simulink library "FMLibrary_v2"  (R2016b)
settings: Solver=ode45  StartTime=0.0  StopTime=10.0  RelTol=1e-3
undefined symbols (not defined in the file or in its folder): ActuatorStruct, drivePeakCurrent, IdxJoint, JointPositionGuardMax_rad, JointPositionGuardMin_rad, Lb, Lf, Lu, motorTorqueConstant, RobotStruct, sampleTime, transmissionRatio
undefined symbols (not defined in the file): JointAbsoluteEncoderCounts_rev
libraries: simulink x23, VariousBlocksLibrary x10, FM_Library x8, FMLibrary_v2 x5, simulink_extras x1
(part 1 of 2)
settings Model: Creator=niekbeckers  LastModifiedBy=niekbeckers
settings DataIOCC: LimitDataPoints=on  SaveFormat=Array
settings OptimizationCC: BlockReduction=off  BooleanDataType=off  LifeSpan=inf
settings DebuggingCC: SaveWithParameterizedLinksMsg=none  UnderspecifiedInitializationDetection=Classic  MergeDetectMultiDrivingBlocksExec=none  SignalResolutionControl=TryResolveAllWithWarning  StrictBusMsg=Warning  SFUnexpectedBacktrackingDiag=warning  SFNoUnconditionalDefaultTransitionDiag=warning  SFExecutionAtInitializationDiag=none
settings HardwareCC: ProdBitPerPointer=32  ProdBitPerSizeT=32  ProdBitPerPtrDiffT=32  ProdLargestAtomicFloat=None  ProdIntDivRoundTo=Undefined  ProdEndianess=Unspecified  ProdWordSize=32  ProdHWDeviceType=32-bit Generic  TargetUnknown=on
settings ModelReferenceCC: PropagateSignalLabelsOutOfModel=off
settings GRTTargetCC: TargetLangStandard=C89/C90 (ANSI)  GeneratePreprocessorConditionals=Disable all
settings ConfigComp: CovMetricSettings=dw  CovHtmlReporting=on  CovSaveCumulativeToWorkspaceVar=on  CovSaveSingleToWorkspaceVar=on  CovExternalEMLEnable=off  CovSFcnEnable=off

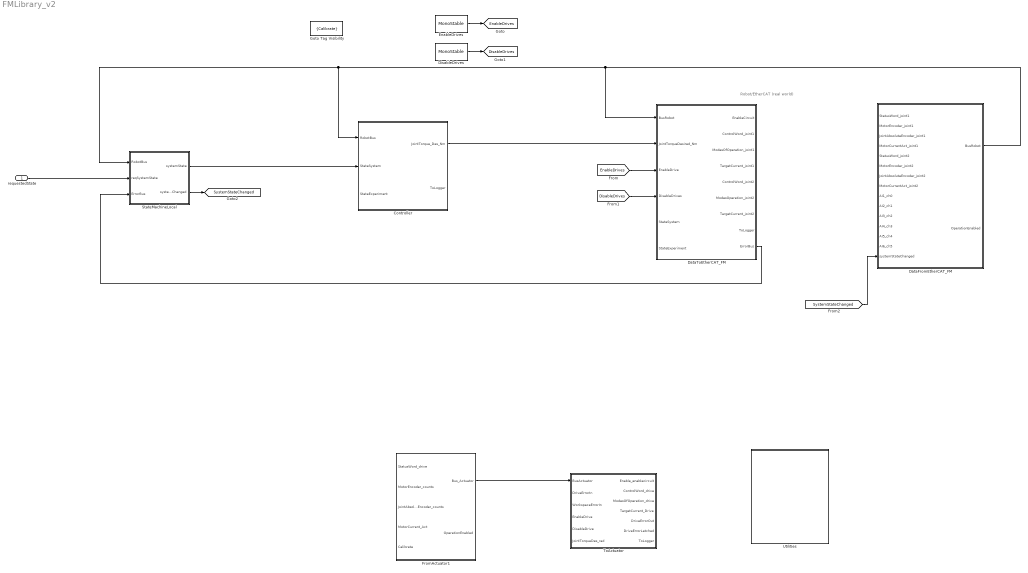
== system FMLibrary_v2 ==
  note: Robot/EtherCAT (real world)
  requestedState : Inport
  Controller : Subsystem
  DataFromEtherCAT_FM : Subsystem
  DataToEtherCAT_FM : Subsystem
  DisableDrives : FM_Library/MonoStable  Value=0  OutMin=[]  OutMax=[]  OutDataTypeStr=Inherit: Inherit from 'Constant value'
  EnableDrives : FM_Library/MonoStable  Value=0  OutMin=[]  OutMax=[]  OutDataTypeStr=Inherit: Inherit from 'Constant value'
  FromActuator1 : Subsystem  mask{ActuatorStruct=RobotStruct.ActuatorStruct}
      mask prompts: ActuatorStruct "Actuator Struct"
  Goto Tag Visibility : GotoTagVisibility  GotoTag=Calibrate
  StateMachineLocal : Subsystem
  ToActuator : Subsystem  mask{ActuatorStruct=RobotStruct.Actuator1}
      mask prompts: ActuatorStruct "Actuator Struct"
  Utilities : Subsystem
  tag scope: DisableDrives=global, EnableDrives=global, SystemStateChanged=global
  wires:
  FromActuator1/1(Bus_Actuator) -> ToActuator/1(BusActuator)
  [EnableDrives] -> DataToEtherCAT_FM/3(EnableDrive)
  [DisableDrives] -> DataToEtherCAT_FM/4(DisableDrives)
  DisableDrives/1 -> [DisableDrives]
  EnableDrives/1 -> [EnableDrives]
  Controller/1(JointTorque_Des_Nm) -> DataToEtherCAT_FM/2(JointTorqueDesired_Nm)
  requestedState/1 -> StateMachineLocal/2(reqSystemState)
  StateMachineLocal/1(systemState) -> Controller/2(StateSystem)
  DataFromEtherCAT_FM/1(BusRobot) -> DataToEtherCAT_FM/1(BusRobot), Controller/1(RobotBus), StateMachineLocal/1(RobotBus)
  DataToEtherCAT_FM/9(ErrorBus) -> StateMachineLocal/3(ErrorBus)
  StateMachineLocal/2(systemStateChanged) -> [SystemStateChanged]
  [SystemStateChanged] -> DataFromEtherCAT_FM/15(systemStateChanged)

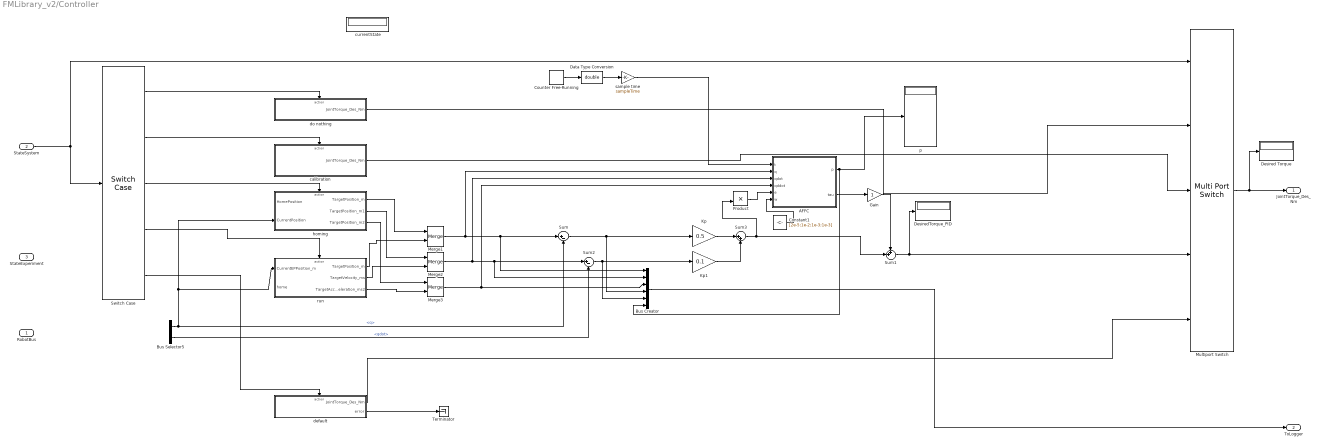
== system FMLibrary_v2/Controller ==
  RobotBus : Inport
  StateSystem : Inport  Port=2
  StateExperiment : Inport  Port=3
  AFFC : MATLAB Function  TreatAsAtomicUnit=on
  Bus Creator : BusCreator  Inputs=6
  Bus Selector5 : BusSelector  OutputSignals=q,qdot
  Constant1 : Constant  Value=[2e-5;1e-2;1e-3;1e-3]
  Counter Free-Running : simulink/Sources/Counter Free-Running  NumBits=32  tsamp=-1
  Data Type Conversion : DataTypeConversion  OutDataTypeStr=double
  Desired Torque : Display
  DesiredTorque_PID : Display
  Gain : Gain
  Kp : Gain  Gain=0.5
  Kp1 : Gain  Gain=0.1
  Merge1 : Merge  InitialOutput=[0;0]
  Merge2 : Merge  InitialOutput=[0;0]
  Merge3 : Merge  InitialOutput=[0;0]
  Multiport Switch : MultiPortSwitch  DataPortOrder=Specify indices  Inputs=4  DataPortIndices={[0,1,201,202,-1],[2],[3,301,4],5}
  Product : Product
  Sum : Sum  Inputs=|+-
  Sum1 : Sum  Inputs=++|
  Sum2 : Sum  Inputs=|+-
  Sum3 : Sum  Inputs=|++
  Switch Case : SwitchCase  CaseConditions={[0,1,201,202,-1],[2],[3,301],4}
  Terminator : Terminator
  calibration : Subsystem  TreatAsAtomicUnit=on
  currentState : Display
  default : Subsystem  TreatAsAtomicUnit=on
  do nothing : Subsystem  TreatAsAtomicUnit=on
  homing : Subsystem
  p : Display
  run : Subsystem
  sample time : Gain  Gain=sampleTime
  JointTorque_Des_Nm : Outport
  ToLogger : Outport  Port=2
  wires:
  Switch Case/2 -> calibration/Action
  Switch Case/1 -> do nothing/Action
  do nothing/1(JointTorque_Des_Nm) -> Multiport Switch/2
  calibration/1(JointTorque_Des_Nm) -> Multiport Switch/3
  default/1(JointTorque_Des_Nm) -> Multiport Switch/5
  Switch Case/5 -> default/Action
  Multiport Switch/1 -> Desired Torque/1, JointTorque_Des_Nm/1
  Switch Case/4 -> run/Action
  Sum/1 -> Bus Creator/4, Kp/1
  homing/1(TargetPosition_m) -> Merge1/1
  Merge1/1 -> AFFC/2(q), Bus Creator/1, Sum/1
  run/1(TargetPosition_m) -> Merge1/2
  Switch Case/3 -> homing/Action
  StateSystem/1 -> Multiport Switch/1, Switch Case/1
  Bus Selector5/1 -> run/1(CurrentEPPosition_m), homing/2(CurrentPosition), Sum/2  "<q>"
  Sum3/1 -> Product/2, Sum1/2
  Sum1/1 -> DesiredTorque_PID/1, Multiport Switch/4
  Gain/1 -> Sum1/1
  run/2(TargetVelocity_ms) -> Merge2/2
  Sum2/1 -> Kp1/1, Bus Creator/5
  Bus Selector5/2 -> Sum2/2  "<qdot>"
  run/3(TargetAcceleration_ms2) -> Merge3/2
  homing/2(TargetPosition_m1) -> Merge2/1
  Merge2/1 -> AFFC/3(qdot), Bus Creator/2, Sum2/1
  homing/3(TargetPosition_m2) -> Merge3/1
  Merge3/1 -> AFFC/4(qddot), Bus Creator/3
  Bus Creator/1 -> ToLogger/1
  default/2(error) -> Terminator/1
  Kp/1 -> Sum3/1
  Kp1/1 -> Sum3/2
  AFFC/1(p) -> Bus Creator/6, p/1
  Data Type Conversion/1 -> sample time/1
  Counter Free-Running/1 -> Data Type Conversion/1
  sample time/1 -> AFFC/1(t)
  Product/1 -> AFFC/5(e)
  Constant1/1 -> AFFC/6(w)
  AFFC/2(tau) -> Gain/1

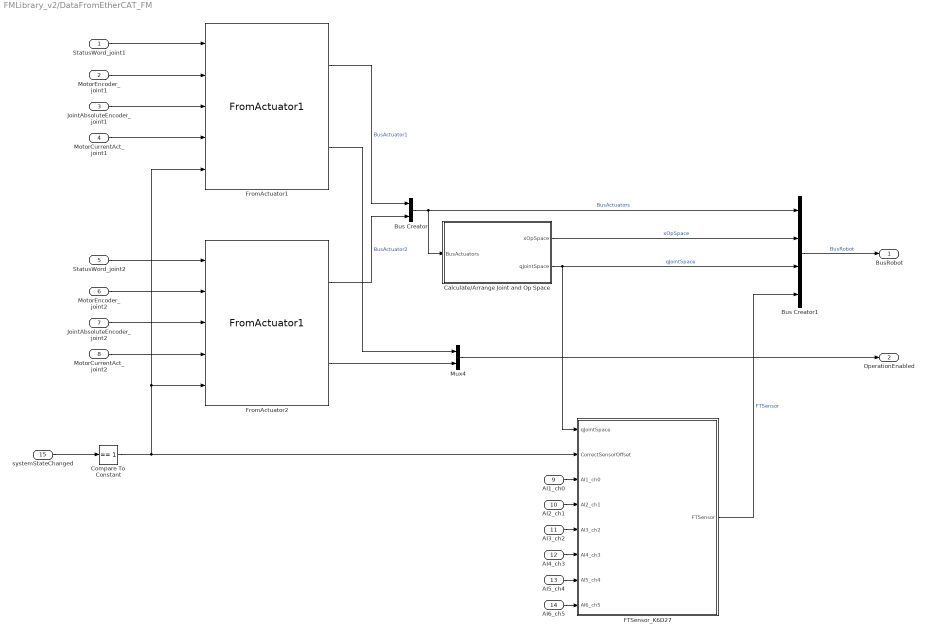
== system FMLibrary_v2/DataFromEtherCAT_FM ==
  StatusWord_joint1 : Inport
  MotorEncoder_joint1 : Inport  Port=2
  JointAbsoluteEncoder_joint1 : Inport  Port=3
  MotorCurrentAct_joint1 : Inport  Port=4
  StatusWord_joint2 : Inport  Port=5
  MotorEncoder_joint2 : Inport  Port=6
  "JointAbsoluteEncoder_joint2 " : Inport  Port=7
  MotorCurrentAct_joint2 : Inport  Port=8
  AI1_ch0 : Inport  Port=9  OutDataTypeStr=int16
  AI2_ch1 : Inport  Port=10  OutDataTypeStr=int16
  AI3_ch2 : Inport  Port=11  OutDataTypeStr=int16
  AI4_ch3 : Inport  Port=12  OutDataTypeStr=int16
  AI5_ch4 : Inport  Port=13  OutDataTypeStr=int16
  AI6_ch5 : Inport  Port=14  OutDataTypeStr=int16
  systemStateChanged : Inport  Port=15
  Bus Creator : BusCreator  Inputs=2
  Bus Creator1 : BusCreator  Inputs=4
  Calculate/Arrange Joint and Op Space : Subsystem
  Compare To Constant : simulink/Logic and Bit Operations/Compare To Constant  relop===  const=1  OutDataTypeStr=boolean
  FTSensor_K6D27 : Subsystem  mask{FTSensorStruct=RobotStruct.FTSensor}
      mask prompts: FTSensorStruct "Struct for force torque sensor"
  FromActuator1 : FMLibrary_v2/Utilities/FromActuator1  ActuatorStruct=RobotStruct.ActuatorStruct
  FromActuator2 : FMLibrary_v2/Utilities/FromActuator1  ActuatorStruct=RobotStruct.ActuatorStruct
  Mux4 : Mux  Inputs=2
  BusRobot : Outport
  OperationEnabled : Outport  Port=2
  wires:
  FromActuator1/1 -> Bus Creator/1  "BusActuator1"
  FromActuator2/1 -> Bus Creator/2  "BusActuator2"
  FromActuator1/2 -> Mux4/1
  Mux4/1 -> OperationEnabled/1
  FromActuator2/2 -> Mux4/2
  MotorEncoder_joint1/1 -> FromActuator1/2
  StatusWord_joint1/1 -> FromActuator1/1
  JointAbsoluteEncoder_joint1/1 -> FromActuator1/3
  MotorCurrentAct_joint1/1 -> FromActuator1/4
  MotorEncoder_joint2/1 -> FromActuator2/2
  StatusWord_joint2/1 -> FromActuator2/1
  "JointAbsoluteEncoder_joint2 "/1 -> FromActuator2/3
  MotorCurrentAct_joint2/1 -> FromActuator2/4
  Bus Creator/1 -> Calculate/Arrange Joint and Op Space/1(BusActuators), Bus Creator1/1  "BusActuators"
  Bus Creator1/1 -> BusRobot/1  "BusRobot"
  Calculate/Arrange Joint and Op Space/1(xOpSpace) -> Bus Creator1/2  "xOpSpace"
  Calculate/Arrange Joint and Op Space/2(qJointSpace) -> FTSensor_K6D27/1(qJointSpace), Bus Creator1/3  "qJointSpace"
  systemStateChanged/1 -> Compare To Constant/1
  AI1_ch0/1 -> FTSensor_K6D27/3(AI1_ch0)
  AI2_ch1/1 -> FTSensor_K6D27/4(AI2_ch1)
  AI3_ch2/1 -> FTSensor_K6D27/5(AI3_ch2)
  AI4_ch3/1 -> FTSensor_K6D27/6(AI4_ch3)
  AI5_ch4/1 -> FTSensor_K6D27/7(AI5_ch4)
  AI6_ch5/1 -> FTSensor_K6D27/8(AI6_ch5)
  FTSensor_K6D27/1(FTSensor) -> Bus Creator1/4  "FTSensor"
  Compare To Constant/1 -> FromActuator2/5, FromActuator1/5, FTSensor_K6D27/2(CorrectSensorOffset)

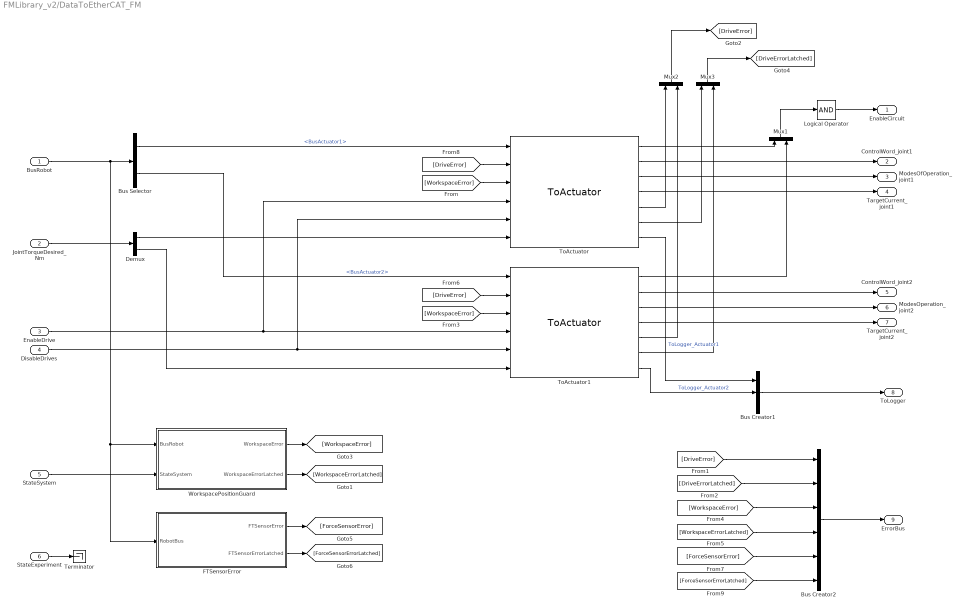
== system FMLibrary_v2/DataToEtherCAT_FM ==
  BusRobot : Inport
  JointTorqueDesired_Nm : Inport  Port=2
  EnableDrive : Inport  Port=3
  DisableDrives : Inport  Port=4
  StateSystem : Inport  Port=5
  StateExperiment : Inport  Port=6
  Bus Creator1 : BusCreator  Inputs=3
  Bus Creator2 : BusCreator  Inputs=6
  Bus Selector : BusSelector  OutputSignals=BusActuators.BusActuator1,BusActuators.BusActuator2
  Demux : Demux  Outputs=2
  FTSensorError : Subsystem
  Logical Operator : Logic  Inputs=1  AllPortsSameDT=off  OutDataTypeStr=boolean
  Mux1 : Mux  Inputs=2
  Mux2 : Mux  Inputs=2
  Mux3 : Mux  Inputs=2
  Terminator : Terminator
  ToActuator : FMLibrary_v2/ToActuator  ActuatorStruct=RobotStruct.Actuator1
  ToActuator1 : FMLibrary_v2/ToActuator  ActuatorStruct=RobotStruct.Actuator1
  WorkspacePositionGuard : Subsystem
  EnableCircuit : Outport
  ControlWord_joint1 : Outport  Port=2
  ModesOfOperation_joint1 : Outport  Port=3
  TargetCurrent_joint1 : Outport  Port=4
  ControlWord_joint2 : Outport  Port=5
  ModesOperation_joint2 : Outport  Port=6
  TargetCurrent_joint2 : Outport  Port=7
  ToLogger : Outport  Port=8
  ErrorBus : Outport  Port=9
  wires:
  ToActuator/5 -> Mux2/1
  ToActuator1/5 -> Mux2/2
  Mux2/1 -> [DriveError]
  ToActuator/6 -> Mux3/1
  ToActuator1/6 -> Mux3/2
  [DriveError] -> ToActuator/2
  Mux1/1 -> Logical Operator/1
  ToActuator/1 -> Mux1/1
  ToActuator1/1 -> Mux1/2
  ToActuator/2 -> ControlWord_joint1/1
  ToActuator/3 -> ModesOfOperation_joint1/1
  ToActuator1/2 -> ControlWord_joint2/1
  ToActuator/4 -> TargetCurrent_joint1/1
  ToActuator1/4 -> TargetCurrent_joint2/1
  ToActuator1/3 -> ModesOperation_joint2/1
  Logical Operator/1 -> EnableCircuit/1
  ToActuator/7 -> Bus Creator1/1  "ToLogger_Actuator1"
  Demux/2 -> ToActuator1/6
  JointTorqueDesired_Nm/1 -> Demux/1
  Demux/1 -> ToActuator/6
  BusRobot/1 -> FTSensorError/1(RobotBus), WorkspacePositionGuard/1(BusRobot), Bus Selector/1
  Bus Selector/2 -> ToActuator1/1  "<BusActuator2>"
  Bus Selector/1 -> ToActuator/1  "<BusActuator1>"
  Bus Creator1/1 -> ToLogger/1
  ToActuator1/7 -> Bus Creator1/2  "ToLogger_Actuator2"
  WorkspacePositionGuard/2(WorkspaceErrorLatched) -> [WorkspaceErrorLatched]
  WorkspacePositionGuard/1(WorkspaceError) -> [WorkspaceError]
  [WorkspaceError] -> ToActuator/3
  DisableDrives/1 -> ToActuator/5, ToActuator1/5
  EnableDrive/1 -> ToActuator/4, ToActuator1/4
  [DriveError] -> ToActuator1/2
  [WorkspaceError] -> ToActuator1/3
  Mux3/1 -> [DriveErrorLatched]
  Bus Creator2/1 -> ErrorBus/1
  [DriveError] -> Bus Creator2/1
  [DriveErrorLatched] -> Bus Creator2/2
  [WorkspaceError] -> Bus Creator2/3
  [WorkspaceErrorLatched] -> Bus Creator2/4
  StateSystem/1 -> WorkspacePositionGuard/2(StateSystem)
  FTSensorError/1(FTSensorError) -> [ForceSensorError]
  FTSensorError/2(FTSensorErrorLatched) -> [ForceSensorErrorLatched]
  [ForceSensorError] -> Bus Creator2/5
  [ForceSensorErrorLatched] -> Bus Creator2/6
  StateExperiment/1 -> Terminator/1

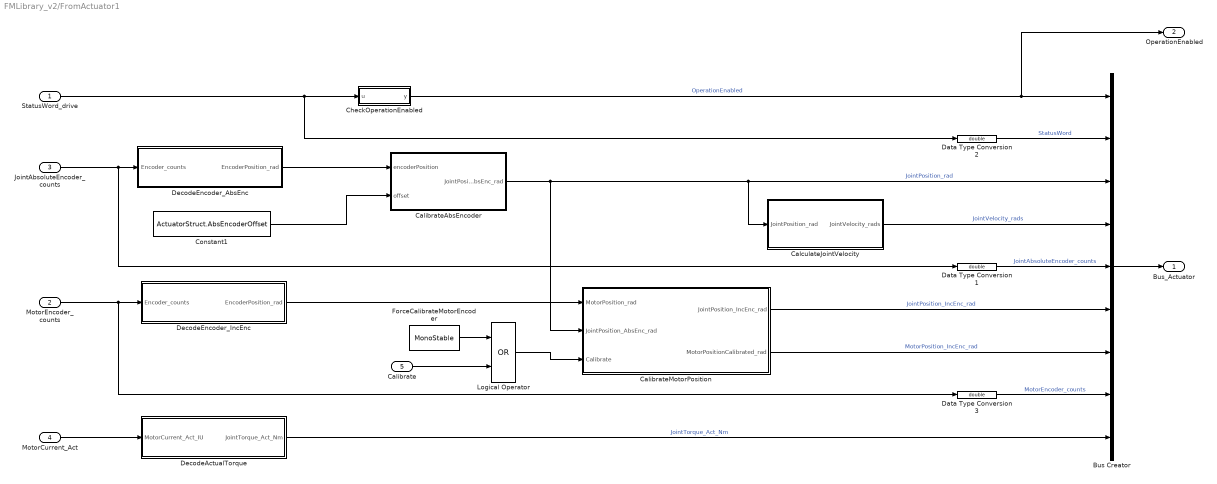
== system FMLibrary_v2/FromActuator1 ==
  StatusWord_drive : Inport
  MotorEncoder_counts : Inport  Port=2
  JointAbsoluteEncoder_counts : Inport  Port=3
  MotorCurrent_Act : Inport  Port=4
  Calibrate : Inport  Port=5
  Bus Creator : BusCreator  Inputs=9
  CalculateJointVelocity : Subsystem
  CalibrateAbsEncoder : MATLAB Function  TreatAsAtomicUnit=on
  "CalibrateMotorPosition    " : MATLAB Function  TreatAsAtomicUnit=on  mask{gearboxRatio=ActuatorStruct.transmissionRatio}
      mask prompts: gearboxRatio "Transmission ratio (e.g. -8) [-]"
  CheckOperationEnabled : MATLAB Function  TreatAsAtomicUnit=on
  Constant1 : Constant  Value=ActuatorStruct.AbsEncoderOffset
  Data Type Conversion1 : DataTypeConversion  OutDataTypeStr=double
  Data Type Conversion2 : DataTypeConversion  OutDataTypeStr=double
  Data Type Conversion3 : DataTypeConversion  OutDataTypeStr=double
  DecodeActualTorque : MATLAB Function  TreatAsAtomicUnit=on  mask(DecodeActualTorque){transmissionRatio=ActuatorStruct.transmissionRatio, motorTorqueConstant=ActuatorStruct.motorTorqueConstant, drivePeakCurrent=ActuatorStruct.drivePeakCurrent}
      mask prompts: transmissionRatio "Transmission ratio (e.g. -8) [-]"; motorTorqueConstant "Motor torque constant [Nm/A]"; drivePeakCurrent "Motor drive peak current Ipeak [A]"
      mask help:
      | Decode Actual Torque value returned from the actuator (motor drive and motor) to torque on the joint (after transmission).
      |
      | Note: due to the way the transmission is set up and the positive motor axis (clockwise is positive as seen from the motor front), there is no need to account for sign change in motor torque or encoder position.
  DecodeEncoder_AbsEnc : MATLAB Function  TreatAsAtomicUnit=on  mask(DecodeEncoder){EncoderCounts_rev=ActuatorStruct.JointAbsoluteEncoderCounts_rev}
      mask prompts: EncoderCounts_rev "Motor encoder increments per revolution (e.g., 8192)"
      mask help: Decode the encoder counts to encoder position in radians
  DecodeEncoder_IncEnc : MATLAB Function  TreatAsAtomicUnit=on  mask(DecodeEncoder){EncoderCounts_rev=ActuatorStruct.MotorEncoderCounts_rev}
      mask prompts: EncoderCounts_rev "Motor encoder increments per revolution (e.g., 8192)"
      mask help: Decode the encoder counts to encoder position in radians
  ForceCalibrateMotorEncoder : FM_Library/MonoStable  Value=0  OutMin=[]  OutMax=[]  OutDataTypeStr=Inherit: Inherit from 'Constant value'
  Logical Operator : Logic  Operator=OR  AllPortsSameDT=off  OutDataTypeStr=boolean
  Bus_Actuator : Outport
  OperationEnabled : Outport  Port=2
  wires:
  Calibrate/1 -> Logical Operator/2
  CalculateJointVelocity/1(JointVelocity_rads) -> Bus Creator/4  "JointVelocity_rads"
  DecodeEncoder_AbsEnc/1(EncoderPosition_rad) -> CalibrateAbsEncoder/1(encoderPosition)
  "CalibrateMotorPosition    "/2(MotorPositionCalibrated_rad) -> Bus Creator/7  "MotorPosition_IncEnc_rad"
  DecodeActualTorque/1(JointTorque_Act_Nm) -> Bus Creator/9  "JointTorque_Act_Nm"
  StatusWord_drive/1 -> Data Type Conversion2/1, CheckOperationEnabled/1(u)
  DecodeEncoder_IncEnc/1(EncoderPosition_rad) -> "CalibrateMotorPosition    "/1(MotorPosition_rad)
  MotorCurrent_Act/1 -> DecodeActualTorque/1(MotorCurrent_Act_IU)
  CheckOperationEnabled/1(y) -> OperationEnabled/1, Bus Creator/1  "OperationEnabled"
  JointAbsoluteEncoder_counts/1 -> Data Type Conversion1/1, DecodeEncoder_AbsEnc/1(Encoder_counts)
  "CalibrateMotorPosition    "/1(JointPosition_IncEnc_rad) -> Bus Creator/6  "JointPosition_IncEnc_rad"
  Data Type Conversion1/1 -> Bus Creator/5  "JointAbsoluteEncoder_counts"
  Data Type Conversion2/1 -> Bus Creator/2  "StatusWord"
  CalibrateAbsEncoder/1(JointPosition_AbsEnc_rad) -> "CalibrateMotorPosition    "/2(JointPosition_AbsEnc_rad), CalculateJointVelocity/1(JointPosition_rad), Bus Creator/3  "JointPosition_rad"
  MotorEncoder_counts/1 -> DecodeEncoder_IncEnc/1(Encoder_counts), Data Type Conversion3/1
  Data Type Conversion3/1 -> Bus Creator/8  "MotorEncoder_counts"
  Bus Creator/1 -> Bus_Actuator/1
  Logical Operator/1 -> "CalibrateMotorPosition    "/3(Calibrate)
  Constant1/1 -> CalibrateAbsEncoder/2(offset)
  ForceCalibrateMotorEncoder/1 -> Logical Operator/1

== system FMLibrary_v2/StateMachineLocal ==
  RobotBus : Inport
  reqSystemState : Inport  Port=2
  ErrorBus : Inport  Port=3
  Bus Selector : BusSelector  OutputSignals=xOpSpace.x,xOpSpace.xdot
  Constant : Constant  Value=RobotStruct.HomeLocationSize
  Constant1 : Constant  Value=RobotStruct.HomeLocation
  Detect Change1 : simulink/Logic and Bit Operations/Detect Change  vinit=0  InputProcessing=Inherited  OutDataTypeStr=boolean
  MATLAB Function : MATLAB Function  TreatAsAtomicUnit=on
  SystemLocalStateMachine : Stateflow chart  TreatAsAtomicUnit=on
  systemState : Outport
  systemStateChanged : Outport  Port=2
  wires:
  reqSystemState/1 -> SystemLocalStateMachine/1(reqSystemState)
  SystemLocalStateMachine/1(currentSystemState) -> systemState/1, MATLAB Function/2(state), Detect Change1/1
  ErrorBus/1 -> SystemLocalStateMachine/2(error)
  Detect Change1/1 -> MATLAB Function/1(stateChanged)
  MATLAB Function/1(systemStateChanged) -> systemStateChanged/1
  Constant/1 -> SystemLocalStateMachine/6(homeLocationSize)
  Constant1/1 -> SystemLocalStateMachine/5(HomePosition)
  RobotBus/1 -> Bus Selector/1
  Bus Selector/1 -> SystemLocalStateMachine/3(x)  "<x>"
  Bus Selector/2 -> SystemLocalStateMachine/4(xdot)  "<xdot>"

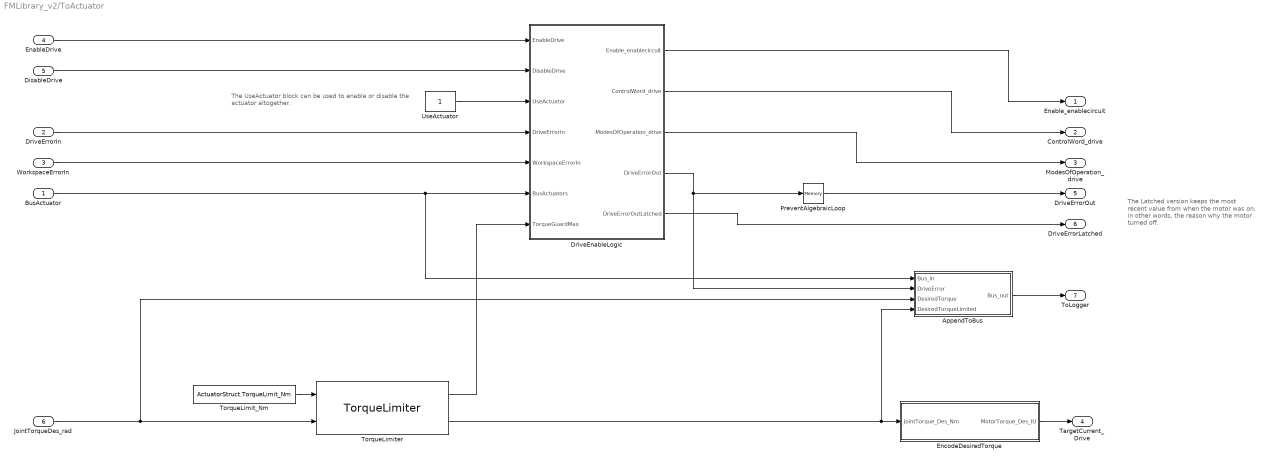
== system FMLibrary_v2/ToActuator ==
  note: The UseActuator block can be used to enable or disable the actuator altogether.
  note: The Latched version keeps the most recent value from when the motor was on; in other words, the reason why the motor turned off.
  BusActuator : Inport
  DriveErrorIn : Inport  Port=2
  WorkspaceErrorIn : Inport  Port=3
  EnableDrive : Inport  Port=4
  DisableDrive : Inport  Port=5
  JointTorqueDes_rad : Inport  Port=6
  AppendToBus : Subsystem
  DriveEnableLogic : Subsystem
  EncodeDesiredTorque : MATLAB Function  TreatAsAtomicUnit=on  mask(EncodeDesiredTorque){transmissionRatio=ActuatorStruct.transmissionRatio, motorTorqueConstant=ActuatorStruct.motorTorqueConstant, drivePeakCurrent=ActuatorStruct.drivePeakCurrent}
      mask prompts: transmissionRatio "Transmission ratio (e.g. -8) [-]"; motorTorqueConstant "Motor torque constant [Nm/A]"; drivePeakCurrent "Motor drive peak current [A]"
      mask help:
      | Encode desired torque at the joint to torque to be produced by the motor.
      |
      | Note: due to the way the transmission is set up and the positive motor axis (clockwise is positive as seen from the motor front), there is no need to account for sign change in motor torque or encoder position.
  PreventAlgebraicLoop : Memory
  TorqueLimit_Nm : Constant  Value=ActuatorStruct.TorqueLimit_Nm
  TorqueLimiter : FM_Library/TorqueLimiter
  UseActuator : Constant  OutDataTypeStr=double
      settings: OpenFcn=|
      | b = get_param(gcb,'value');
      | if (strcmp(b,'1')),
      |   set_param (gcb,'value','0');
      | else
      |   set_param(gcb,'value','1');
      | end;
  Enable_enablecircuit : Outport
  ControlWord_drive : Outport  Port=2
  ModesOfOperation_drive : Outport  Port=3
  TargetCurrent_Drive : Outport  Port=4
  DriveErrorOut : Outport  Port=5
  DriveErrorLatched : Outport  Port=6
  ToLogger : Outport  Port=7
  wires:
  UseActuator/1 -> DriveEnableLogic/3(UseActuator)
  AppendToBus/1(Bus_out) -> ToLogger/1
  PreventAlgebraicLoop/1 -> DriveErrorOut/1
  DriveErrorIn/1 -> DriveEnableLogic/4(DriveErrorIn)
  DriveEnableLogic/4(DriveErrorOut) -> PreventAlgebraicLoop/1, AppendToBus/2(DriveError)
  DisableDrive/1 -> DriveEnableLogic/2(DisableDrive)
  EnableDrive/1 -> DriveEnableLogic/1(EnableDrive)
  BusActuator/1 -> AppendToBus/1(Bus_in), DriveEnableLogic/6(BusActuators)
  EncodeDesiredTorque/1(MotorTorque_Des_IU) -> TargetCurrent_Drive/1
  DriveEnableLogic/2(ControlWord_drive) -> ControlWord_drive/1
  DriveEnableLogic/3(ModesOfOperation_drive) -> ModesOfOperation_drive/1
  TorqueLimit_Nm/1 -> TorqueLimiter/1
  DriveEnableLogic/5(DriveErrorOutLatched) -> DriveErrorLatched/1
  TorqueLimiter/2 -> EncodeDesiredTorque/1(JointTorque_Des_Nm), AppendToBus/4(DesiredTorqueLimited)
  TorqueLimiter/1 -> DriveEnableLogic/7(TorqueGuardMax)
  JointTorqueDes_rad/1 -> TorqueLimiter/2, AppendToBus/3(DesiredTorque)
  DriveEnableLogic/1(Enable_enablecircuit) -> Enable_enablecircuit/1
  WorkspaceErrorIn/1 -> DriveEnableLogic/5(WorkspaceErrorIn)

== system FMLibrary_v2/Utilities ==
  Boolean : Constant  Value=false  OutDataTypeStr=boolean
      settings: OpenFcn=|
      | b = get_param(gcb,'value');
      | if (strcmp(b,'true')),
      |   set_param (gcb,'value','false');
      | else
      |   set_param(gcb,'value','true');
      | end;
  Boolean1 : Constant  OutDataTypeStr=double
      settings: OpenFcn=|
      | b = get_param(gcb,'value');
      | if (strcmp(b,'1')),
      |   set_param (gcb,'value','0');
      | else
      |   set_param(gcb,'value','1');
      | end;
  CrossFade : Subsystem
  Cycloid : Subsystem
  DecodeActualTorque : MATLAB Function  TreatAsAtomicUnit=on  mask(DecodeActualTorque){transmissionRatio=transmissionRatio, motorTorqueConstant=motorTorqueConstant, drivePeakCurrent=drivePeakCurrent}
      mask prompts: transmissionRatio "Transmission ratio (e.g. -8) [-]"; motorTorqueConstant "Motor torque constant [Nm/A]"; drivePeakCurrent "Motor drive peak current Ipeak [A]"
      mask help:
      | Decode Actual Torque value returned from the actuator (motor drive and motor) to torque on the joint (after transmission).
      |
      | Note: due to the way the transmission is set up and the positive motor axis (clockwise is positive as seen from the motor front), there is no need to account for sign change in motor torque or encoder position.
  DecodeEncoder : MATLAB Function  TreatAsAtomicUnit=on  mask(DecodeEncoder){EncoderCounts_rev=JointAbsoluteEncoderCounts_rev}
      mask prompts: EncoderCounts_rev "Motor encoder increments per revolution (e.g., 8192)"
      mask help: Decode the encoder counts to encoder position in radians
  EncodeDesiredTorque : MATLAB Function  TreatAsAtomicUnit=on  mask(EncodeDesiredTorque){transmissionRatio=transmissionRatio, motorTorqueConstant=motorTorqueConstant, drivePeakCurrent=drivePeakCurrent}
      mask prompts: transmissionRatio "Transmission ratio (e.g. -8) [-]"; motorTorqueConstant "Motor torque constant [Nm/A]"; drivePeakCurrent "Motor drive peak current [A]"
      mask help:
      | Encode desired torque at the joint to torque to be produced by the motor.
      |
      | Note: due to the way the transmission is set up and the positive motor axis (clockwise is positive as seen from the motor front), there is no need to account for sign change in motor torque or encoder position.
  EndstopAndSafety : Subsystem
  FOAW : MATLAB Function  TreatAsAtomicUnit=on
  FilterFourthOrder : Subsystem
  Latch : Subsystem  mask{ic=0}
      mask prompts: ic "Initial Condition"
  LatchRising : Subsystem  mask{ic=0}
      mask prompts: ic "Initial Condition"
  MonoStable : Constant  Value=0
      settings: OpenFcn=set_param(gcb,'Value','1');tname = ['toggletimer_' gcb];delete(timerfind('name',tname));t = timer('timerfcn', ['set_param(''',gcb,''',''Value'',''0'')'],'executionmode','singleshot','startdelay',1,'name',tname);start(t);
      mask Display: fprintf('PushToTrigger\n%s',get_param(gcb,'value'))
  Stopwatch : Subsystem
  TorqueLimiter : Subsystem

== system FMLibrary_v2/Controller/calibration ==
  Action Port : ActionPort  InitializeStates=reset
  Constant3 : Constant  Value=[0;0]
  JointTorque_Des_Nm : Outport  InitialOutput=[0;0]
  wires:
  Constant3/1 -> JointTorque_Des_Nm/1

== system FMLibrary_v2/Controller/default ==
  Action Port : ActionPort  InitializeStates=reset
  Constant1 : Constant  OutDataTypeStr=boolean
  Constant3 : Constant  Value=[0;0]
  JointTorque_Des_Nm : Outport  InitialOutput=[0;0]
  error : Outport  Port=2  OutDataTypeStr=boolean
  wires:
  Constant3/1 -> JointTorque_Des_Nm/1
  Constant1/1 -> error/1

== system FMLibrary_v2/Controller/do nothing ==
  Action Port : ActionPort  InitializeStates=reset
  Constant3 : Constant  Value=[0;0]
  JointTorque_Des_Nm : Outport
  wires:
  Constant3/1 -> JointTorque_Des_Nm/1

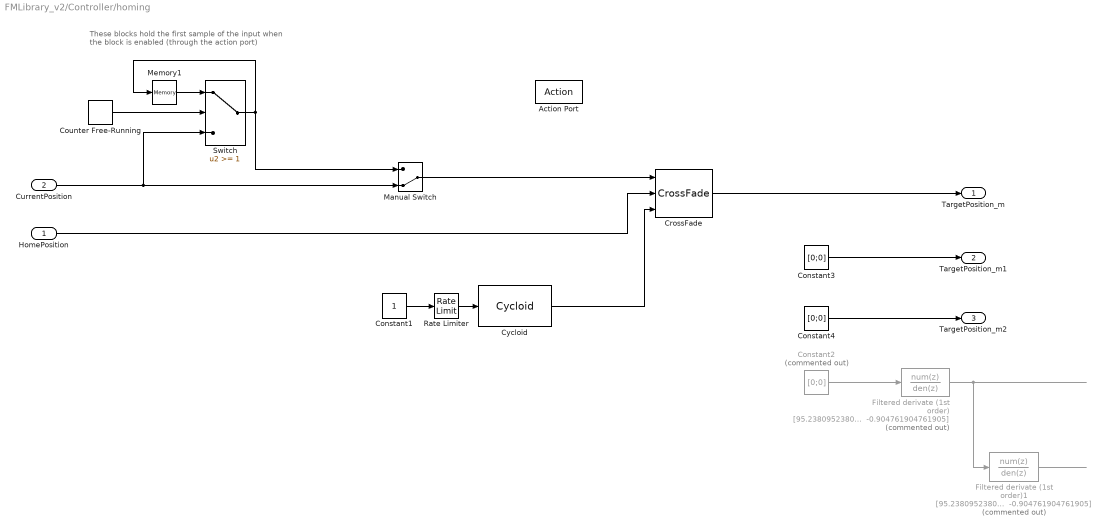
== system FMLibrary_v2/Controller/homing ==
  note: These blocks hold the first sample of the input
      | when the block is enabled (through the action port)
  HomePosition : Inport
  CurrentPosition : Inport  Port=2
  Action Port : ActionPort  InitializeStates=reset
  Constant1 : Constant
  Constant2 : Constant  Commented=on  Value=[0;0]
  Constant3 : Constant  Value=[0;0]
  Constant4 : Constant  Value=[0;0]
  Counter Free-Running : simulink/Sources/Counter Free-Running  NumBits=32  tsamp=-1
  CrossFade : VariousBlocksLibrary/Various/CrossFade
  Cycloid : VariousBlocksLibrary/Various/Cycloid
  Filtered derivate (1st order) : DiscreteTransferFcn  Commented=on  Numerator=[95.238095238095241 -95.238095238095241]  Denominator="[1.000000000000000  -0.904761904761905]"
  Filtered derivate (1st order)1 : DiscreteTransferFcn  Commented=on  Numerator=[95.238095238095241 -95.238095238095241]  Denominator="[1.000000000000000  -0.904761904761905]"
  Manual Switch : ManualSwitch  CurrentSetting=0
  Memory1 : Memory
  Rate Limiter : RateLimiter  RisingSlewLimit=0.2  FallingSlewLimit=-0.2  SampleTimeMode=inherited
  Switch : Switch  Threshold=1
  TargetPosition_m : Outport  InitialOutput=[0;0]
  TargetPosition_m1 : Outport  Port=2  InitialOutput=[0;0]
  TargetPosition_m2 : Outport  Port=3  InitialOutput=[0;0]
  wires:
  CurrentPosition/1 -> Manual Switch/2, Switch/3
  HomePosition/1 -> CrossFade/2
  Cycloid/1 -> CrossFade/3
  Rate Limiter/1 -> Cycloid/1
  Constant1/1 -> Rate Limiter/1
  Switch/1 -> Memory1/1, Manual Switch/1
  Counter Free-Running/1 -> Switch/2
  Memory1/1 -> Switch/1
  Manual Switch/1 -> CrossFade/1
  CrossFade/1 -> TargetPosition_m/1
  Filtered derivate (1st order)/1 -> Filtered derivate (1st order)1/1
  Filtered derivate (1st order)1/1 -> ?
  Constant2/1 -> Filtered derivate (1st order)/1
  Constant3/1 -> TargetPosition_m1/1
  Constant4/1 -> TargetPosition_m2/1

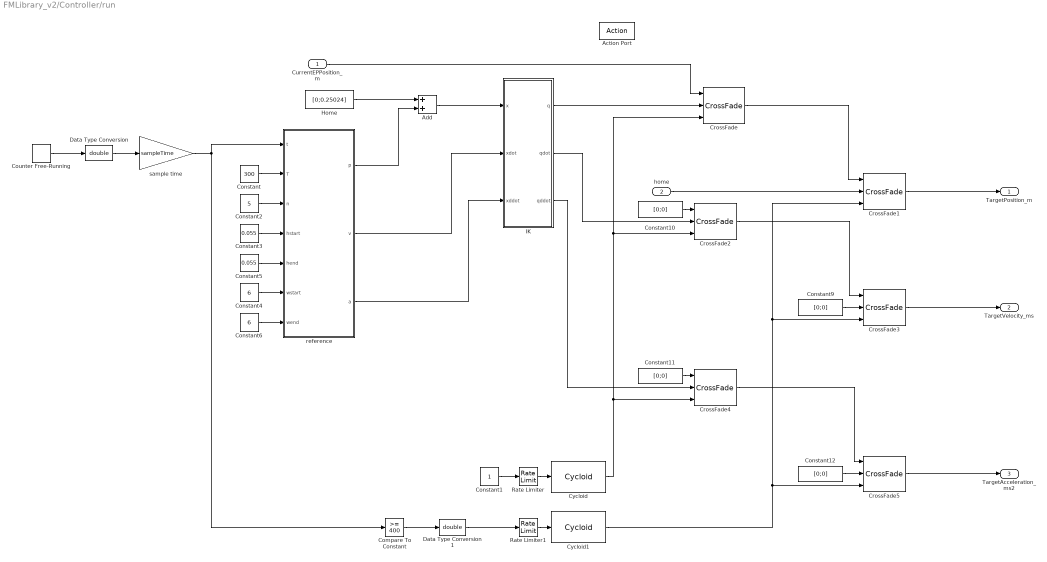
== system FMLibrary_v2/Controller/run ==
  CurrentEPPosition_m : Inport
  home : Inport  Port=2
  Action Port : ActionPort  InitializeStates=reset
  Add : Sum
  Compare To Constant : simulink/Logic and Bit Operations/Compare To Constant  relop=>=  const=400  OutDataTypeStr=boolean
  Constant : Constant  Value=300
  Constant1 : Constant
  Constant{9..12} (4 alike) : Constant  Value=[0;0]
  Constant2 : Constant  Value=5
  Constant3 : Constant  Value=0.055
  Constant4 : Constant  Value=6
  Constant5 : Constant  Value=0.055
  Constant6 : Constant  Value=6
  Counter Free-Running : simulink/Sources/Counter Free-Running  NumBits=32  tsamp=-1
  CrossFade{,1..5} (6 alike) : VariousBlocksLibrary/Various/CrossFade
  Cycloid : VariousBlocksLibrary/Various/Cycloid
  Cycloid1 : VariousBlocksLibrary/Various/Cycloid
  Data Type Conversion : DataTypeConversion  OutDataTypeStr=double
  Data Type Conversion1 : DataTypeConversion  OutDataTypeStr=double
  "Home " : Constant  Value=[0;0.25024]
  IK : MATLAB Function  TreatAsAtomicUnit=on
  Rate Limiter : RateLimiter  RisingSlewLimit=0.25  FallingSlewLimit=-0.15  SampleTimeMode=inherited
  Rate Limiter1 : RateLimiter  RisingSlewLimit=0.2  FallingSlewLimit=-0.2  SampleTimeMode=inherited
  reference : MATLAB Function  TreatAsAtomicUnit=on
  sample time : Gain  Gain=sampleTime
  TargetPosition_m : Outport
  TargetVelocity_ms : Outport  Port=2
  TargetAcceleration_ms2 : Outport  Port=3
  wires:
  Cycloid/1 -> CrossFade2/3, CrossFade/3, CrossFade4/3
  Constant1/1 -> Rate Limiter/1
  Rate Limiter/1 -> Cycloid/1
  CurrentEPPosition_m/1 -> CrossFade/1
  CrossFade1/1 -> TargetPosition_m/1
  CrossFade/1 -> CrossFade1/1
  home/1 -> CrossFade1/2
  Compare To Constant/1 -> Data Type Conversion1/1
  Rate Limiter1/1 -> Cycloid1/1
  Cycloid1/1 -> CrossFade5/3, CrossFade3/3, CrossFade1/3
  CrossFade3/1 -> TargetVelocity_ms/1
  CrossFade2/1 -> CrossFade3/1
  Constant9/1 -> CrossFade3/2
  Constant10/1 -> CrossFade2/1
  CrossFade4/1 -> CrossFade5/1
  Constant12/1 -> CrossFade5/2
  Constant11/1 -> CrossFade4/1
  CrossFade5/1 -> TargetAcceleration_ms2/1
  Data Type Conversion/1 -> sample time/1
  Counter Free-Running/1 -> Data Type Conversion/1
  sample time/1 -> Compare To Constant/1, reference/1(t)
  Constant/1 -> reference/2(T)
  Constant2/1 -> reference/3(n)
  Constant5/1 -> reference/5(hend)
  Constant3/1 -> reference/4(hstart)
  Constant6/1 -> reference/7(wend)
  Constant4/1 -> reference/6(wstart)
  reference/3(a) -> IK/3(xddot)
  reference/2(v) -> IK/2(xdot)
  reference/1(p) -> Add/2
  Add/1 -> IK/1(x)
  "Home "/1 -> Add/1
  IK/2(qdot) -> CrossFade2/2
  IK/1(q) -> CrossFade/2
  IK/3(qddot) -> CrossFade4/2
  Data Type Conversion1/1 -> Rate Limiter1/1

== system FMLibrary_v2/DataFromEtherCAT_FM/Calculate//Arrange Joint and Op Space ==
  note: Here all angles of the parallel mechanism are calculated
      | based on the endpoint position, though this may still lead to incorrect
      | estimations of the internal angles (e.g. it is possible that on of the elbows
      | has gone through a singular position already). So perhaps I should also include
      | a different way of calculating the internal angles
  BusActuators : Inport
  Bus Creator1 : BusCreator  Inputs=3
  Bus Creator2 : BusCreator  Inputs=3
  Bus Selector : BusSelector  OutputSignals=BusActuator1.JointPosition_rad,BusActuator2.JointPosition_rad  OutputAsBus=on
  Bus Selector1 : BusSelector  OutputSignals=BusActuator1.JointVelocity_rads,BusActuator2.JointVelocity_rads  OutputAsBus=on
  Bus Selector2 : BusSelector  OutputSignals=BusActuator1.JointPosition_rad,BusActuator2.JointPosition_rad,BusActuator1.JointVelocity_rads,BusActuator2.JointVelocity_rads
  Ground : Ground
  IK all joints : MATLAB Function  TreatAsAtomicUnit=on
  Mux : Mux  Inputs=2
  Mux1 : Mux  Inputs=2
  Terminator1 : Terminator
  Terminator2 : Terminator
  forward kinematics : Subsystem
  xOpSpace : Outport
  qJointSpace : Outport  Port=2
  wires:
  forward kinematics/5(Jdot) -> Terminator2/1
  forward kinematics/3(xddot) -> Terminator1/1
  forward kinematics/2(xdot) -> Bus Creator1/2  "xdot"
  Bus Selector/1 -> forward kinematics/1(JointPosition_rad)
  forward kinematics/1(x) -> IK all joints/1(x), Bus Creator1/1  "x"
  Bus Creator1/1 -> xOpSpace/1  "OpSpace"
  forward kinematics/4(J) -> Bus Creator1/3  "jacobian"
  Bus Selector1/1 -> forward kinematics/2(JointVelocity_rads)
  Ground/1 -> forward kinematics/3(JointAcceleration_rads2)
  Bus Creator2/1 -> qJointSpace/1  "JointSpace"
  BusActuators/1 -> Bus Selector1/1, Bus Selector2/1, Bus Selector/1
  Mux/1 -> Bus Creator2/1  "q"
  Bus Selector2/1 -> Mux/1  "<JointPosition_rad>"
  Bus Selector2/2 -> Mux/2  "<JointPosition_rad>"
  Bus Selector2/3 -> Mux1/1  "<JointVelocity_rads>"
  Bus Selector2/4 -> Mux1/2  "<JointVelocity_rads>"
  Mux1/1 -> Bus Creator2/2  "qdot"
  IK all joints/1(q_all) -> Bus Creator2/3  "qall"

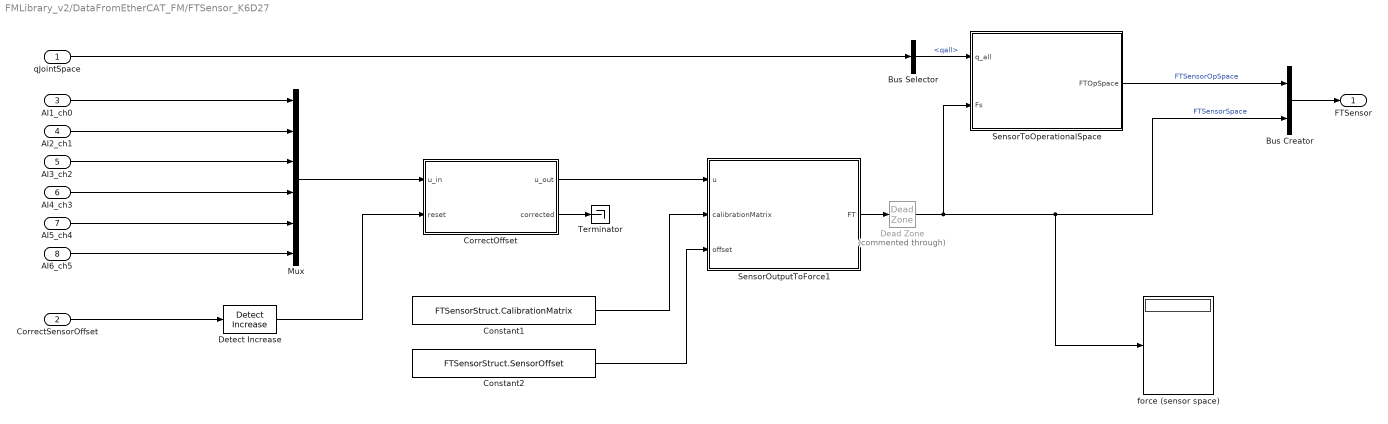
== system FMLibrary_v2/DataFromEtherCAT_FM/FTSensor_K6D27 ==
  qJointSpace : Inport
  CorrectSensorOffset : Inport  Port=2
  AI1_ch0 : Inport  Port=3  OutDataTypeStr=int16
  AI2_ch1 : Inport  Port=4  OutDataTypeStr=int16
  AI3_ch2 : Inport  Port=5  OutDataTypeStr=int16
  AI4_ch3 : Inport  Port=6  OutDataTypeStr=int16
  AI5_ch4 : Inport  Port=7  OutDataTypeStr=int16
  AI6_ch5 : Inport  Port=8  OutDataTypeStr=int16
  Bus Creator : BusCreator  Inputs=2
  Bus Selector : BusSelector  OutputSignals=qall
  Constant1 : Constant  Value=FTSensorStruct.CalibrationMatrix
  Constant2 : Constant  Value=FTSensorStruct.SensorOffset
  CorrectOffset : MATLAB Function  TreatAsAtomicUnit=on
  Dead Zone : DeadZone  Commented=through  LowerValue=-0.05  UpperValue=0.05  SaturateOnIntegerOverflow=on
  Detect Increase : simulink/Logic and Bit Operations/Detect Increase  vinit=0.0  InputProcessing=Inherited  OutDataTypeStr=boolean
  Mux : Mux  Inputs=6
  SensorOutputToForce1 : MATLAB Function  TreatAsAtomicUnit=on
  SensorToOperationalSpace : MATLAB Function  TreatAsAtomicUnit=on
  Terminator : Terminator
  force (sensor space) : Display
  FTSensor : Outport
  wires:
  qJointSpace/1 -> Bus Selector/1
  AI2_ch1/1 -> Mux/2
  AI1_ch0/1 -> Mux/1
  CorrectOffset/1(u_out) -> SensorOutputToForce1/1(u)
  Mux/1 -> CorrectOffset/1(u_in)
  CorrectSensorOffset/1 -> Detect Increase/1
  Detect Increase/1 -> CorrectOffset/2(reset)
  SensorOutputToForce1/1(FT) -> Dead Zone/1
  Bus Selector/1 -> SensorToOperationalSpace/1(q_all)  "<qall>"
  AI6_ch5/1 -> Mux/6
  AI5_ch4/1 -> Mux/5
  AI4_ch3/1 -> Mux/4
  AI3_ch2/1 -> Mux/3
  CorrectOffset/2(corrected) -> Terminator/1
  Dead Zone/1 -> Bus Creator/2, force (sensor space)/1, SensorToOperationalSpace/2(Fs)  "FTSensorSpace"
  Constant1/1 -> SensorOutputToForce1/2(calibrationMatrix)
  Constant2/1 -> SensorOutputToForce1/3(offset)
  Bus Creator/1 -> FTSensor/1
  SensorToOperationalSpace/1(FTOpSpace) -> Bus Creator/1  "FTSensorOpSpace"

== system FMLibrary_v2/DataToEtherCAT_FM/FTSensorError ==
  RobotBus : Inport
  AvoidAlgebraicLoop : Memory
  Bus Selector1 : BusSelector  OutputSignals=FTSensor.FTSensorSpace
  Constant : Constant  Value=RobotStruct.MaxAllowableForcesTorqueSensor
  CreateSingleErrorValue : FMLibrary_v2/DataToEtherCAT_FM/WorkspacePositionGuard/CreateSingleErrorValue
  Detect Change : simulink/Logic and Bit Operations/Detect Change  vinit=0  InputProcessing=Inherited  OutDataTypeStr=boolean
  FTSensorLastError : Display
  LatchRising : FM_Library/LatchRising  ic=0
  MATLAB Function : MATLAB Function  TreatAsAtomicUnit=on
  ShowFTSensorErrorLatched : Display
  FTSensorError : Outport
  FTSensorErrorLatched : Outport  Port=2
  wires:
  Detect Change/1 -> LatchRising/Trigger
  AvoidAlgebraicLoop/1 -> FTSensorError/1, Detect Change/1, LatchRising/1
  LatchRising/1 -> FTSensorErrorLatched/1, ShowFTSensorErrorLatched/1
  CreateSingleErrorValue/1 -> AvoidAlgebraicLoop/1
  RobotBus/1 -> Bus Selector1/1
  Bus Selector1/1 -> MATLAB Function/1(ForcesTorques)  "<FTSensorSpace>"
  MATLAB Function/1(e) -> CreateSingleErrorValue/1, FTSensorLastError/1
  Constant/1 -> MATLAB Function/2(MaxForcesTorques)

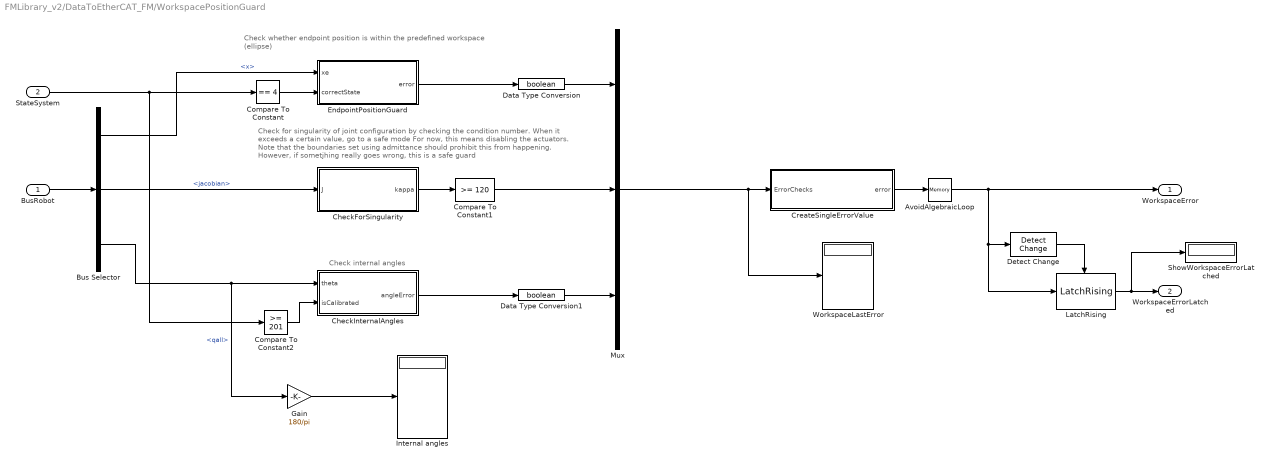
== system FMLibrary_v2/DataToEtherCAT_FM/WorkspacePositionGuard ==
  note: Check internal angles
  note: Check whether endpoint position is within the predefined workspace
      | (ellipse)
  note: Check for singularity of joint configuration by checking
      | the condition number. When it exceeds a certain value, go to a safe mode
      | For now, this means disabling the actuators.
      | Note that the boundaries set using admittance should prohibit this from happening.
      | However, if sometjhing really goes wrong, this is a safe guard
  BusRobot : Inport
  StateSystem : Inport  Port=2
  AvoidAlgebraicLoop : Memory
  Bus Selector : BusSelector  OutputSignals=xOpSpace.x,xOpSpace.jacobian,qJointSpace.qall
  CheckForSingularity : MATLAB Function  TreatAsAtomicUnit=on
  CheckInternalAngles : MATLAB Function  TreatAsAtomicUnit=on
  Compare To Constant : simulink/Logic and Bit Operations/Compare To Constant  relop===  const=4  OutDataTypeStr=boolean
  Compare To Constant1 : simulink/Logic and Bit Operations/Compare To Constant  relop=>=  const=120  OutDataTypeStr=boolean
  Compare To Constant2 : simulink/Logic and Bit Operations/Compare To Constant  relop=>=  const=201  OutDataTypeStr=boolean
  CreateSingleErrorValue : Subsystem
  Data Type Conversion : DataTypeConversion  OutDataTypeStr=boolean
  Data Type Conversion1 : DataTypeConversion  OutDataTypeStr=boolean
  Detect Change : simulink/Logic and Bit Operations/Detect Change  vinit=0  InputProcessing=Inherited  OutDataTypeStr=boolean
  EndpointPositionGuard : MATLAB Function  TreatAsAtomicUnit=on
  Gain : Gain  Gain=180/pi
  Internal angles : Display
  LatchRising : FM_Library/LatchRising  ic=0
  Mux : Mux  Inputs=3
  ShowWorkspaceErrorLatched : Display
  WorkspaceLastError : Display
  WorkspaceError : Outport
  WorkspaceErrorLatched : Outport  Port=2
  wires:
  CheckForSingularity/1(kappa) -> Compare To Constant1/1
  Mux/1 -> WorkspaceLastError/1, CreateSingleErrorValue/1(ErrorChecks)
  EndpointPositionGuard/1(error) -> Data Type Conversion/1
  BusRobot/1 -> Bus Selector/1
  Bus Selector/1 -> EndpointPositionGuard/1(xe)  "<x>"
  Bus Selector/3 -> Gain/1, CheckInternalAngles/1(theta)  "<qall>"
  CheckInternalAngles/1(angleError) -> Data Type Conversion1/1
  LatchRising/1 -> ShowWorkspaceErrorLatched/1, WorkspaceErrorLatched/1
  Compare To Constant1/1 -> Mux/2
  Data Type Conversion/1 -> Mux/1
  Data Type Conversion1/1 -> Mux/3
  CreateSingleErrorValue/1(error) -> AvoidAlgebraicLoop/1
  Detect Change/1 -> LatchRising/Trigger
  AvoidAlgebraicLoop/1 -> Detect Change/1, LatchRising/1, WorkspaceError/1
  Compare To Constant/1 -> EndpointPositionGuard/2(correctState)
  Compare To Constant2/1 -> CheckInternalAngles/2(isCalibrated)
  Gain/1 -> Internal angles/1
  Bus Selector/2 -> CheckForSingularity/1(J)  "<jacobian>"
  StateSystem/1 -> Compare To Constant2/1, Compare To Constant/1

== system FMLibrary_v2/FromActuator1/CalculateJointVelocity ==
  JointPosition_rad : Inport
  Discrete Derivative : simulink/Discrete/Discrete Derivative  Commented=on  gainval=1.0  ICPrevScaledInput=0.0  InputProcessing=Inherited  OutMin=[]  OutMax=[]  OutDataType=fixdt(1, 16)  OutScaling=2^-10  DoSatur=off
  FOAW : MATLAB Function  TreatAsAtomicUnit=on
  Filter1 : FM_Library/FilterFourthOrder/Filter1  Commented=on  sampleTime=sampleTime
  Omega1 : Constant  Commented=on  Value=2*pi*100  OutDataTypeStr=double
  encoder noise : Constant  Value=ActuatorStruct.FOAWNoiseLevel
  JointVelocity_rads : Outport
  wires:
  JointPosition_rad/1 -> FOAW/1(x)
  Filter1/1 -> ?
  Discrete Derivative/1 -> Filter1/1
  Omega1/1 -> Filter1/2
  FOAW/1(xdot) -> JointVelocity_rads/1
  encoder noise/1 -> FOAW/2(noise)

== system FMLibrary_v2/ToActuator/AppendToBus ==
  Bus_in : Inport
  DriveError : Inport  Port=2
  DesiredTorque : Inport  Port=3
  DesiredTorqueLimited : Inport  Port=4
  Bus Creator : BusCreator  Inputs=13
  Bus Selector2 : BusSelector  OutputSignals=OperationEnabled,StatusWord,JointPosition_rad,JointVelocity_rads,MotorEncoder_counts,MotorPosition_IncEnc_rad,JointPosition_IncEnc_rad,JointAbsoluteEncoder_counts,JointTorque_Act_Nm
  Data Type Conversion : DataTypeConversion  OutDataTypeStr=double
  Bus_out : Outport
  wires:
  Bus Selector2/6 -> Bus Creator/6  "<MotorPosition_IncEnc_rad>"
  Bus Selector2/8 -> Bus Creator/8  "<JointAbsoluteEncoder_counts>"
  Bus Selector2/7 -> Bus Creator/7  "<JointPosition_IncEnc_rad>"
  Bus Selector2/5 -> Bus Creator/5  "<MotorEncoder_counts>"
  Bus Selector2/4 -> Bus Creator/4  "<JointVelocity_rads>"
  Bus Selector2/3 -> Bus Creator/3  "<JointPosition_rad>"
  Bus Selector2/2 -> Bus Creator/2  "<StatusWord>"
  Bus Selector2/1 -> Bus Creator/1  "<OperationEnabled>"
  DesiredTorqueLimited/1 -> Bus Creator/11  "DesiredTorqueLimited_Nm"
  DesiredTorque/1 -> Bus Creator/10  "DesiredTorque_Nm"
  Data Type Conversion/1 -> Bus Creator/12  "DriveError"
  DriveError/1 -> Data Type Conversion/1
  Bus_in/1 -> Bus Selector2/1
  Bus Creator/1 -> Bus_out/1
  Bus Selector2/9 -> Bus Creator/9  "<JointTorque_Act_Nm>"

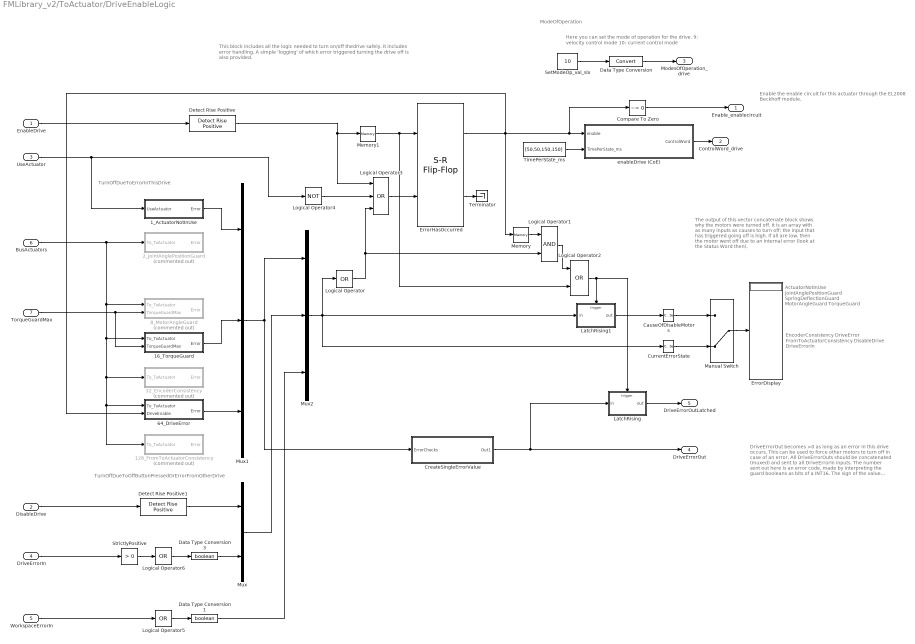
== system FMLibrary_v2/ToActuator/DriveEnableLogic ==
  note: Enable the enable circuit for this actuator through the EL2008
      | Beckhoff module.
  note: ModeOfOperation
  note: ActuatorNotInUse
      | JointAnglePositionGuard
      | SpringDeflectionGuard
      | MotorAngleGuard
      | TorqueGuard
  note: EncoderConsistency
      | DriveError
      | FromToActuatorConsistency
      | DisableDrive
      | DriveErrorIn
  note: DriveErrorOut becomes >0 as long as an error in this drive occurs. This can be used to force other motors to turn off in case of an error.
      | All DriveErrorOuts should be concatenated (muxed)  and sent to all DriveErrorIn inputs. The number sent out here is an error code, made by interpreting the guard booleans as bits of a INT16.
      | The sign of the value indicates:
      | >=0: UseActuator=true
      | <0: UseActuator = False
  note: TurnOffDueToOffButtonPressedOrErrorFromOtherDrive
  note: TurnOffDueToErrorInThisDrive
  note: This block includes all the logic needed to turn on/off thedrive safely. It includes error handling. A simple 'logging' of which error triggered turning the drive off is also provided.
  note: The output of this vector concatenate block shows why the motors were turned off. It is an array with as many inputs as causes to turn off; the input that has triggered going off is high. If all are low, then the motor went off due to an internal error (look at the Status Word then).
  note: Here you can set the mode of operation for the drive.
      | 9: velocity control mode
      | 10: current control mode
  EnableDrive : Inport
  DisableDrive : Inport  Port=2
  UseActuator : Inport  Port=3
  DriveErrorIn : Inport  Port=4
  WorkspaceErrorIn : Inport  Port=5
  BusActuators : Inport  Port=6
  TorqueGuardMax : Inport  Port=7
  128_FromToActuatorConsistency : Subsystem  Commented=on
  16_TorqueGuard : Subsystem
  1_ActuatorNotInUse : Subsystem
  2_JointAnglePositionGuard : Subsystem  Commented=on
  32_EncoderConsistency : Subsystem  Commented=on
  64_DriveError : Subsystem
  8_MotorAngleGuard : Subsystem  Commented=on
  CauseOfDisableMotors : Concatenate  NumInputs=1
  Compare To Zero : simulink/Logic and Bit Operations/Compare To Zero  relop=~=  OutDataTypeStr=boolean
  CreateSingleErrorValue : Subsystem
  CurrentErrorState : Concatenate  NumInputs=1
  Data Type Conversion : DataTypeConversion
  Data Type Conversion1 : DataTypeConversion  OutDataTypeStr=boolean
  Data Type Conversion3 : DataTypeConversion  OutDataTypeStr=boolean
  Detect Rise Positive : simulink/Logic and Bit Operations/Detect Rise Positive  vinit=0  InputProcessing=Inherited  OutDataTypeStr=boolean
  Detect Rise Positive1 : simulink/Logic and Bit Operations/Detect Rise Positive  vinit=0  InputProcessing=Inherited  OutDataTypeStr=boolean
  ErrorDisplay : Display
  ErrorHasOccurred : simulink_extras/Flip Flops/S-R Flip-Flop  initial_condition=0
  LatchRising : Subsystem  TreatAsAtomicUnit=on
  LatchRising1 : Subsystem  TreatAsAtomicUnit=on
  Logical Operator : Logic  Operator=OR  Inputs=1  AllPortsSameDT=off  OutDataTypeStr=boolean
  Logical Operator1 : Logic  AllPortsSameDT=off  OutDataTypeStr=boolean
  Logical Operator2 : Logic  Operator=OR  AllPortsSameDT=off  OutDataTypeStr=boolean
  Logical Operator3 : Logic  Operator=OR  Inputs=3  AllPortsSameDT=off  OutDataTypeStr=boolean
  Logical Operator4 : Logic  Operator=NOT  Inputs=1  AllPortsSameDT=off  OutDataTypeStr=boolean
  Logical Operator5 : Logic  Operator=OR  Inputs=1  AllPortsSameDT=off  OutDataTypeStr=boolean
  Logical Operator6 : Logic  Operator=OR  Inputs=1  AllPortsSameDT=off  OutDataTypeStr=boolean
  Manual Switch : ManualSwitch  CurrentSetting=0
  Memory : Memory
  Memory1 : Memory
  Mux : Mux  Inputs=2
  Mux1 : Mux  Inputs=3
  Mux2 : Mux  Inputs=3
  SetModeOp_val_slx : Constant  Value=10
  StrictlyPositive : simulink/Logic and Bit Operations/Compare To Zero  relop=>  OutDataTypeStr=boolean
  Terminator : Terminator
  TimePerState_ms : Constant  Value=[50,50,150,150]
  enableDrive (CoE) : MATLAB Function  TreatAsAtomicUnit=on
  Enable_enablecircuit : Outport
  ControlWord_drive : Outport  Port=2
  ModesOfOperation_drive : Outport  Port=3
  DriveErrorOut : Outport  Port=4
  DriveErrorOutLatched : Outport  Port=5
  wires:
  LatchRising/1(out) -> DriveErrorOutLatched/1
  CreateSingleErrorValue/1(Out1) -> DriveErrorOut/1, LatchRising/1(in)
  StrictlyPositive/1 -> Logical Operator6/1
  TorqueGuardMax/1 -> 16_TorqueGuard/2(TorqueGuardMax), 8_MotorAngleGuard/2(TorqueGuardMax)
  LatchRising1/1(out) -> CauseOfDisableMotors/1
  Logical Operator/1 -> Logical Operator3/3, Logical Operator1/2
  SetModeOp_val_slx/1 -> Data Type Conversion/1
  EnableDrive/1 -> Detect Rise Positive/1
  enableDrive (CoE)/1(ControlWord) -> ControlWord_drive/1
  ErrorHasOccurred/1 -> Memory/1, 64_DriveError/2(DriveEnable), Compare To Zero/1, enableDrive (CoE)/1(enable)
  Mux2/1 -> Logical Operator/1, CurrentErrorState/1, LatchRising1/1(in)
  Detect Rise Positive1/1 -> Mux/1
  DisableDrive/1 -> Detect Rise Positive1/1
  ErrorHasOccurred/2 -> Terminator/1
  Data Type Conversion/1 -> ModesOfOperation_drive/1
  CauseOfDisableMotors/1 -> Manual Switch/1
  Memory1/1 -> Logical Operator2/2, ErrorHasOccurred/1
  Memory/1 -> Logical Operator1/1
  Logical Operator2/1 -> LatchRising1/Trigger, LatchRising/Trigger
  CurrentErrorState/1 -> Manual Switch/2
  Logical Operator1/1 -> Logical Operator2/1
  Manual Switch/1 -> ErrorDisplay/1
  Logical Operator3/1 -> ErrorHasOccurred/2
  Detect Rise Positive/1 -> Logical Operator3/1, Memory1/1
  TimePerState_ms/1 -> enableDrive (CoE)/2(TimePerState_ms)
  UseActuator/1 -> 1_ActuatorNotInUse/1(UseActuator), Logical Operator4/1
  DriveErrorIn/1 -> StrictlyPositive/1
  Logical Operator6/1 -> Data Type Conversion3/1
  Mux/1 -> Mux2/2
  BusActuators/1 -> 2_JointAnglePositionGuard/1(To_ToActuator), 8_MotorAngleGuard/1(To_ToActuator), 16_TorqueGuard/1(To_ToActuator), 128_FromToActuatorConsistency/1(To_ToActuator), 64_DriveError/1(To_ToActuator), 32_EncoderConsistency/1(To_ToActuator)
  Logical Operator4/1 -> Logical Operator3/2
  1_ActuatorNotInUse/1(Error) -> Mux1/1
  64_DriveError/1(Error) -> Mux1/3
  16_TorqueGuard/1(Error) -> Mux1/2
  Compare To Zero/1 -> Enable_enablecircuit/1
  Data Type Conversion3/1 -> Mux/2
  Logical Operator5/1 -> Data Type Conversion1/1
  WorkspaceErrorIn/1 -> Logical Operator5/1
  Mux1/1 -> CreateSingleErrorValue/1(ErrorChecks), Mux2/1
  Data Type Conversion1/1 -> Mux2/3

== system FMLibrary_v2/Utilities/CrossFade ==
  In1 : Inport
  In2 : Inport  Port=2
  AmountIn2 : Inport  Port=3
  Add : Sum  Inputs=+-
  Add1 : Sum
  One : Constant
  Product : Product  RndMeth=Zero
  Product1 : Product  RndMeth=Zero
  Saturation : Saturate  UpperLimit=1  LowerLimit=0
  Out : Outport
  wires:
  In1/1 -> Product1/1
  AmountIn2/1 -> Saturation/1
  One/1 -> Add/1
  Saturation/1 -> Product/2, Add/2
  Add/1 -> Product1/2
  Product/1 -> Add1/2
  Product1/1 -> Add1/1
  In2/1 -> Product/1
  Add1/1 -> Out/1

== system FMLibrary_v2/Utilities/Cycloid ==
  note: Given a linear input 0<=in<=1, it gives a cycloid output 0<=out<=1.
      | If In is outside the 0..1 range, it is limited to 0 or 1.
  In : Inport
  Gain1 : Gain  Gain=2*pi
  Gain2 : Gain  Gain=1/(2*pi)
  Saturation : Saturate  UpperLimit=1  LowerLimit=0
  Subtract : Sum  Inputs=+-
  Trigonometric Function : Trigonometry
  Out : Outport
  wires:
  Gain1/1 -> Trigonometric Function/1
  Subtract/1 -> Out/1
  In/1 -> Saturation/1
  Saturation/1 -> Gain1/1, Subtract/1
  Trigonometric Function/1 -> Gain2/1
  Gain2/1 -> Subtract/2

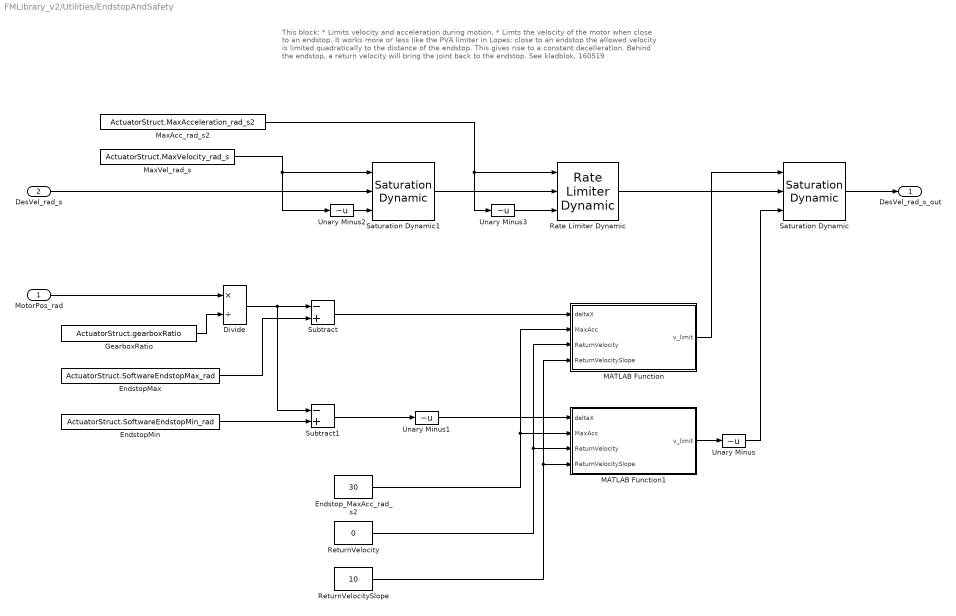
== system FMLibrary_v2/Utilities/EndstopAndSafety ==
  note: This block:
      | * Limits velocity and acceleration during motion,
      | * Limts the velocity of the motor when close to an endstop. It works more or less like the PVA limiter in Lopes: close to an endstop the allowed velocity is limited quadratically to the distance of the endstop. This gives rise to a constant decelleration. Behind the endstop, a return velocity will bring the joint back to the endstop.  See kladblok, 160519
  MotorPos_rad : Inport
  DesVel_rad_s : Inport  Port=2
  Divide : Product  Inputs=*/
  EndstopMax : Constant  Value=ActuatorStruct.SoftwareEndstopMax_rad
  EndstopMin : Constant  Value=ActuatorStruct.SoftwareEndstopMin_rad
  Endstop_MaxAcc_rad_s2 : Constant  Value=30
  GearboxRatio : Constant  Value=ActuatorStruct.gearboxRatio
  MATLAB Function : MATLAB Function  TreatAsAtomicUnit=on
  MATLAB Function1 : MATLAB Function  TreatAsAtomicUnit=on
  MaxAcc_rad_s2 : Constant  Value=ActuatorStruct.MaxAcceleration_rad_s2
  MaxVel_rad_s : Constant  Value=ActuatorStruct.MaxVelocity_rad_s
  Rate Limiter Dynamic : simulink/Discontinuities/Rate Limiter Dynamic
  ReturnVelocity : Constant  Value=0
  ReturnVelocitySlope : Constant  Value=10
  Saturation Dynamic : simulink/Discontinuities/Saturation Dynamic  OutMin=[]  OutMax=[]  OutDataTypeStr=Inherit: Same as second input  OutDataType=fixdt(1, 16)  OutScaling=2^-10  DoSatur=off
  Saturation Dynamic1 : simulink/Discontinuities/Saturation Dynamic  OutMin=[]  OutMax=[]  OutDataTypeStr=Inherit: Same as second input  OutDataType=fixdt(1, 16)  OutScaling=2^-10  DoSatur=off
  Subtract : Sum  Inputs=-+
  Subtract1 : Sum  Inputs=-+
  Unary Minus{,1..3} (4 alike) : UnaryMinus
  DesVel_rad_s_out : Outport
  wires:
  Unary Minus3/1 -> Rate Limiter Dynamic/3
  MaxAcc_rad_s2/1 -> Rate Limiter Dynamic/1, Unary Minus3/1
  Unary Minus2/1 -> Saturation Dynamic1/3
  MaxVel_rad_s/1 -> Saturation Dynamic1/1, Unary Minus2/1
  DesVel_rad_s/1 -> Saturation Dynamic1/2
  Saturation Dynamic1/1 -> Rate Limiter Dynamic/2
  Rate Limiter Dynamic/1 -> Saturation Dynamic/2
  Saturation Dynamic/1 -> DesVel_rad_s_out/1
  MotorPos_rad/1 -> Divide/1
  GearboxRatio/1 -> Divide/2
  Divide/1 -> Subtract1/1, Subtract/1
  EndstopMax/1 -> Subtract/2
  ReturnVelocitySlope/1 -> MATLAB Function1/4(ReturnVelocitySlope), MATLAB Function/4(ReturnVelocitySlope)
  ReturnVelocity/1 -> MATLAB Function1/3(ReturnVelocity), MATLAB Function/3(ReturnVelocity)
  MATLAB Function/1(v_limit) -> Saturation Dynamic/1
  MATLAB Function1/1(v_limit) -> Unary Minus/1
  Subtract1/1 -> Unary Minus1/1
  EndstopMin/1 -> Subtract1/2
  Endstop_MaxAcc_rad_s2/1 -> MATLAB Function1/2(MaxAcc), MATLAB Function/2(MaxAcc)
  Subtract/1 -> MATLAB Function/1(deltaX)
  Unary Minus/1 -> Saturation Dynamic/3
  Unary Minus1/1 -> MATLAB Function1/1(deltaX)

== system FMLibrary_v2/Utilities/FilterFourthOrder ==
  In : Inport
  Omega : Inport  Port=2
  Filter1 : MATLAB Function  TreatAsAtomicUnit=on  mask{sampleTime=sampleTime}
      mask prompts: sampleTime "Sample Time"
  Filter2 : MATLAB Function  TreatAsAtomicUnit=on  mask{sampleTime=sampleTime}
      mask prompts: sampleTime "Sample Time"
  Out : Outport
  wires:
  Filter2/1(y) -> Out/1
  In/1 -> Filter1/1(x)
  Omega/1 -> Filter1/2(OmegaFilter), Filter2/2(OmegaFilter)
  Filter1/1(y) -> Filter2/1(x)
